simulink model "Path_Flyer"  (R2017b)
settings: Solver=VariableStepAuto  StartTime=0.0  StopTime=500  FixedStep=0.01  MaxStep=0.06  RelTol=1e-3  EnableMultiTasking=on
PreLoadFcn:
  | load('Hummingbird_+.mat');
  | load('Hover_Hum.mat');
StartFcn:
  | clear NLGL
  | clear CARROT
  | clear NLGL_ad_2
  | clear CARROT_ad_2
model workspace (MAT data in the model file):
  Sig = Simulink.Signal
  Sig.DataType = 'auto'
  Sig.Dimensions = -1
  Sig.DimensionsMode = 'auto'
  Sig.Complexity = 'auto'
  Sig.SampleTime = -1
  Sig.SamplingMode = 'auto'
undefined symbols (not defined in the file): IC, quadModel
libraries: simulink x18
Description:
  | This is a configurable quadcopter simulation.
  | This Simulink model demonstates position control.
  | 
  | Additional quadcopter modeling and simulation materials available at:
  | github.com/dch33/Quad-Sim
  | 
  | Copyright (C) 2014 D. Hartman, K. Landis, S. Moreno, J. Kim, M. Mehrer
  | 
  | License:
  |     This program is free software: you can redistribute it and/or modify
  |     it under the terms of the GNU LESSER GENERAL PUBLIC LICENSE as published by
  |     the Free Software Foundation, either version 3 of the License, or
  |     (at your option) any later version.
  | 
  |     This program is distributed in the hope that it will be useful,
  |     but WITHOUT ANY WARRANTY; without even the implied warranty of
  |     MERCHANTABILITY or FITNESS FOR A PARTICULAR PURPOSE.  See the
  |     GNU General Public License for more details.
  | 
  |     You should have received a copy of the GNU LESSER GENERAL PUBLIC LICENSE
  |     along with this program.  If not, see <http://www.gnu.org/licenses/>.
settings Model: ModifiedComment=tomeu -- Fri Oct 14 22:31:49 2016 -- Version 1.12  Creator=David Hartman  LastModifiedBy=tomeu
settings Model: ModifiedHistory=|
  | tomeu -- Fri Oct 14 22:31:49 2016 -- Version 1.12
  | 
  | 
  | tomeu -- Fri Oct 14 22:31:49 2016 -- Version 1.12
  | 
  | 
  | tomeu -- Fri Oct 14 00:32:08 2016 -- Version 1.11
  | 
  | 
  | tomeu -- Thu Oct 13 16:50:12 2016 -- Version 1.10
  | 
  | 
  | tomeu -- Thu Oct 13 14:25:45 2016 -- Version 1.9
  | 
  | 
  | tomeu -- Tue Oct 11 16:42:58 2016 -- Version 1.8
  | 
  | 
  | tomeu -- Mon Oct 10 19:40:14 2016 -- Version 1.7
  | 
  | 
  | tomeu -- Mon Oct 10 16:39:20 2016 -- Version 1.6
  | 
  | 
  | davidhartman -- Fri Jun 06 22:59:54 2014 -- Version 1.5
settings DataIOCC: SaveFormat=Array  SignalLogging=off
settings OptimizationCC: DefaultParameterBehavior=Inlined  LifeSpan=inf
settings DebuggingCC: SolverPrmCheckMsg=warning  UniqueDataStoreMsg=warning  AllowSymbolicDim=off  StateNameClashWarn=warning  StrictBusMsg=ErrorOnBusTreatedAsVector  SFUnexpectedBacktrackingDiag=warning  SFNoUnconditionalDefaultTransitionDiag=warning  SFExecutionAtInitializationDiag=none
settings HardwareCC: ProdBitPerPointer=32  ProdBitPerSizeT=32  ProdBitPerPtrDiffT=32  ProdLargestAtomicFloat=None  ProdIntDivRoundTo=Undefined  ProdEndianess=Unspecified  ProdWordSize=32  ProdHWDeviceType=32-bit Generic
settings ModelReferenceCC: PropagateSignalLabelsOutOfModel=off
settings CodeAppCC: StateflowObjectComments=on
settings GRTTargetCC: TargetLangStandard=C89/C90 (ANSI)  GeneratePreprocessorConditionals=Disable all
settings ConfigComp: CovMetricSettings=dw  CovHtmlReporting=on  CovSaveCumulativeToWorkspaceVar=on  CovSaveSingleToWorkspaceVar=on  CovExternalEMLEnable=off

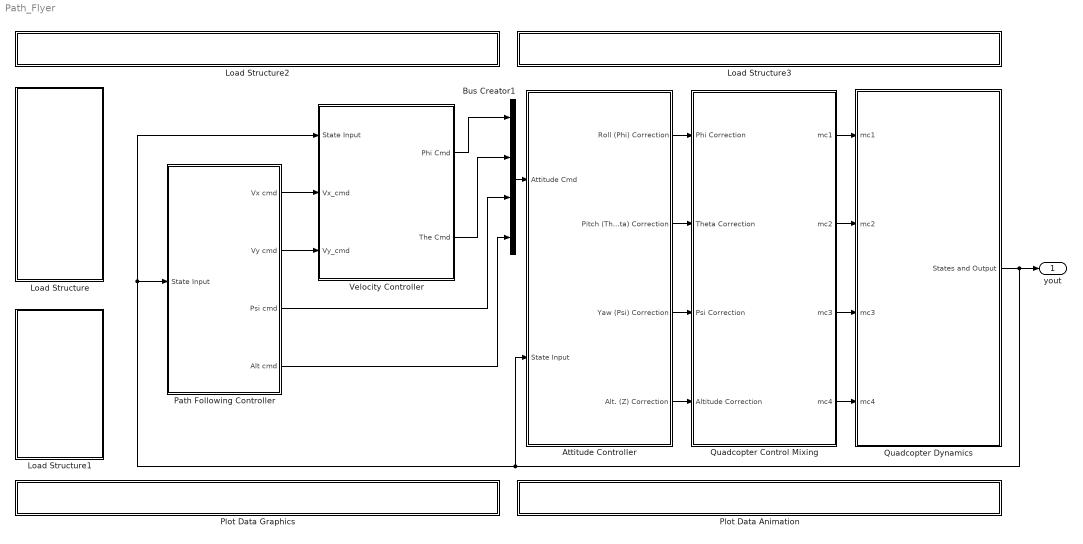
== system Path_Flyer ==
  Attitude Controller : Subsystem
  Bus Creator1 : BusCreator  Inputs=4
  Load Structure : Subsystem
      settings: OpenFcn=|
      | uiopen('load')
      | if ((exist('IC')==1) && (exist('quadModel')==1) && (exist('path')==1))
      | set_param(bdroot, 'SimulationCommand', 'update')
      | end
      mask Display: fprintf('LOAD:\nTimeseries\nPath\nCommands,\nQuadcopter\nModel, Or\nInitial\nConditions');
  Load Structure1 : Subsystem
      settings: OpenFcn=|
      | if (exist('IC')==1 && exist('quadModel')==1 && exist('yout') && exist('tout'))
      | saveSimResults()
      | else
      | msgbox('No Data To Save!')
      | end
      mask Display: fprintf('SAVE:\nSimulation\nResults');
  Load Structure2 : Subsystem
      settings: OpenFcn=|
      | if exist('GUI_Modeling') == 2,
      | run('GUI_Modeling')
      | 
      | else
      | 
      | msgbox('The desired GUI must be first added to MATLABs path.')
      | 
      | end
      mask Display: fprintf('OPEN GUI: Build New \n Model');
  Load Structure3 : Subsystem
      settings: OpenFcn=|
      | if exist('GUI_IC') == 2,
      | run('GUI_IC')
      | 
      | else
      | 
      | msgbox('The desired GUI must be first added to MATLABs path.')
      | 
      | end
      mask Display: fprintf('OPEN GUI: Create Initial \n Conditions');
  Path Following Controller : Subsystem  mask{PF_Algorithm=NLGL, alg_param=1, Adaptive=off, Path_type=Eight-Shaped, Vref=1, A_path=3, gamma_end=1, ZVar=on, Trajplot=on, ErrXplot=off, ErrYplot=off, ErrZplot=off, L2plot=on, YawErrplot=off, Velplot=off, CEffplot=off, AlgParamplot=off, ValueAvgL2=0.18642, ValueAvgYawErr=11.8613, ValueAvgVel=0.97456, ValueAvgCEff=51.0051, ValueTfinal=40.4522}
      mask prompts: alg_param "Algorithm parameter"; Adaptive "Adaptive parameter selection"; Vref "Velocity reference (m/s)"; A_path "Path amplitude (m)"; gamma_end "Path length (turns)"; ZVar "Variable altitude"; Trajplot "3D trajectory"; ErrXplot "Error on X"; ErrYplot "Error on Y"; ErrZplot "Error on Z"; L2plot "Path distance error"; YawErrplot "Yaw angle error"; Velplot "Velocity module"; CEffplot "Control effort"; AlgParamplot "Algorithm parameter"; ValueAvgL2 "Average path distane error (m)"; ValueAvgYawErr "Average absolute yaw error (deg)"; ValueAvgVel "Average absolute velocity (m/s)"; ValueAvgCEff "Average control effort (%)"; ValueTfinal "Total time (s)"
      mask TypeOptions PF_Algorithm: NLGL | Carrot-Chasing
      mask TypeOptions Path_type: Eight-Shaped | Circular | Spiral | Line + Circular
      mask Callback Path_type:
      | Amp_p=str2num(get_param(gcb,'A_path'));
      | load('Hover_Hum.mat');
      | maskStr = get_param(gcb,'Path_type');
      | if strcmp(maskStr,'Eight-Shaped')
      | 	IC.X = IC.X + Amp_p*2;
      |     IC.Psi = IC.Psi + 90;
      | elseif strcmp(maskStr,'Circular')
      | 	IC.X = IC.X + Amp_p;
      |     IC.Psi = IC.Psi + 90;
      | elseif strcmp(maskStr,'Spiral')
      |     IC.Psi = IC.Psi + 90;
      | end
      | 
      | clear maskStr Amp_p;
      mask DialogControl DescGroupVar Prompt: Path Following Control
      mask DialogControl DescTextVar Prompt: This block implements the selected path following algorithm for the desired path command. Parameters such as the velocity of the vehicle, the lenght of the path and the control parameter of the selected algorithm can be changed below.
      mask DialogControl Container5 Prompt: Algorithm
      mask DialogControl Container10 Prompt: Path comand
      mask DialogControl Container3 Prompt: Path Following Evaluation
      mask DialogControl Control4 Prompt: Select which graphs you want to plot and press Run Evaluation button.
      mask DialogControl Container7 Prompt: Plots
      mask DialogControl Container9 Prompt: Results
      mask DialogControl RunEvaluation Prompt: Run Evaluation
      mask DialogControl RunEvaluation Callback:
      | maskStr = get_param(gcb,'Path_type');
      | if strcmp(maskStr,'Eight-Shaped')
      |     path_type = 1;
      | elseif strcmp(maskStr,'Circular')
      |     path_type = 2;
      | elseif strcmp(maskStr,'Spiral')
      |     path_type = 3;
      | elseif strcmp(maskStr,'Line + Circular')
      |     path_type = 4;
      | end
      | 
      | if strcmp(get_param(gcb,'ZVar'),'on')
      |     z_var = 1;
      | else
      |     z_var = 0;
      | end
      | g_end=str2num(get_param(gcb,'gamma_end'));
      | 
      | Amp_path=str2num(get_param(gcb,'A_path'));
      | 
      | Traj_plot = get_param(gcb,'Trajplot');
      | ErrX_plot = get_param(gcb,'ErrXplot');
      | ErrY_plot = get_param(gcb,'ErrYplot');
      | ErrZ_plot = get_param(gcb,'ErrZplot');
      | L2_plot = get_param(gcb,'L2plot');
      | YawErr_plot = get_param(gcb,'YawErrplot');
      | Vel_plot = get_param(gcb,'Velplot');
      | CEff_plot = get_param(gcb,'CEffplot');
      | AlgParam_plot = get_param(gcb,'AlgParamplot');
      | 
      | analyse;
      | 
      | set_param(gcb,'ValueAvgL2',num2str(meanL2_3D));
      | set_param(gcb,'ValueAvgYawErr',num2str(meanAbsYawErr));
      | set_param(gcb,'ValueAvgVel',num2str(meanVel));
      | set_param(gcb,'ValueAvgCEff',num2str(meanCEffort));
      | set_param(gcb,'ValueTfinal',num2str(Tfinal));
      | 
      | clear maskStr path_type Traj_plot ErrX_plot ErrY_plot ErrZ_plot;
      | clear L2_plot YawErr_plot Vel_plot CEff_plot AlgParam_plot g_end z_var;
      | clear meanL2_3D meanAbsYawErr meanVel meanCEffort Tfinal
  Plot Data Animation : Subsystem
      settings: OpenFcn=|
      | if exist('QuadAnim4') == 2,
      |     if exist('yout')
      | 	run('QuadAnim4');
      |     else
      |     msgbox('Simulation must be run before data can be plotted.');
      |     end
      | else                                                                          msgbox('The desired GUI must be first added to MATLABs path.')
      | end
      mask Display: fprintf('OPEN GUI: Flight Animation')
  Plot Data Graphics : Subsystem
      settings: OpenFcn=|
      | if exist('yout')
      | yout = evalin('base', 'yout');
      | tout = evalin('base', 'tout');
      | quadPlots(yout, tout)
      | else
      | msgbox('Simulation must be run before data can be plotted.')
      | end
      mask Display: fprintf('OPEN PLOT: State Data')
  Quadcopter Control Mixing : Subsystem
      mask Display:
      | modelLoaded = evalin('base','exist(''quadModel'',''var'')');
      | if (modelLoaded==1)
      |     if (evalin('base','quadModel.plusConfig'))
      |     fprintf([' \n' ' \n'  'Configuration "+"']);
      |     else if (~evalin('base','quadModel.plusConfig'))
      |         fprintf([' \n' ' \n' 'Configuration "X"']);
      |         end
      |     end
      | else
      |     fprintf([' \n' ' \n'  'Model Not Loaded']);
      | end
  Quadcopter Dynamics : Subsystem
  Velocity Controller : Subsystem
  yout : Outport
  wires:
  Quadcopter Control Mixing/1(mc1) -> Quadcopter Dynamics/1(mc1)
  Quadcopter Control Mixing/2(mc2) -> Quadcopter Dynamics/2(mc2)
  Quadcopter Control Mixing/3(mc3) -> Quadcopter Dynamics/3(mc3)
  Quadcopter Control Mixing/4(mc4) -> Quadcopter Dynamics/4(mc4)
  Attitude Controller/1(Roll (Phi) Correction) -> Quadcopter Control Mixing/1(Phi Correction)
  Attitude Controller/2(Pitch (Theta) Correction) -> Quadcopter Control Mixing/2(Theta Correction)
  Attitude Controller/3(Yaw (Psi) Correction) -> Quadcopter Control Mixing/3(Psi Correction)
  Attitude Controller/4(Alt. (Z) Correction) -> Quadcopter Control Mixing/4(Altitude Correction)
  Quadcopter Dynamics/1(States and Output) -> yout/1, Velocity Controller/1(State Input), Path Following Controller/1(State Input), Attitude Controller/2(State Input)
  Bus Creator1/1 -> Attitude Controller/1(Attitude Cmd)
  Path Following Controller/3(Psi cmd) -> Bus Creator1/3
  Path Following Controller/4(Alt cmd) -> Bus Creator1/4
  Velocity Controller/1(Phi Cmd) -> Bus Creator1/1
  Velocity Controller/2(The Cmd) -> Bus Creator1/2
  Path Following Controller/2(Vy cmd) -> Velocity Controller/3(Vy_cmd)
  Path Following Controller/1(Vx cmd) -> Velocity Controller/2(Vx_cmd)

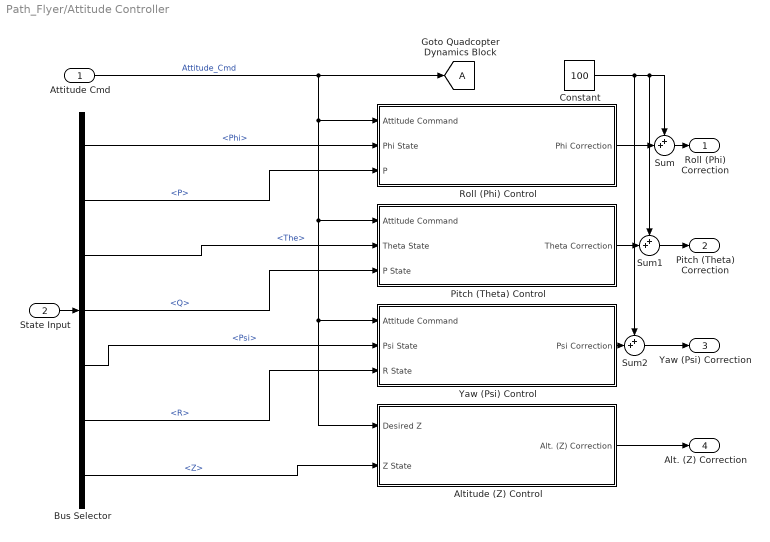
== system Path_Flyer/Attitude Controller ==
  Attitude Cmd : Inport
  State Input : Inport  Port=2
  Altitude (Z) Control : Subsystem  mask{Kpz=2*2, Kiz=1.1*2, Kdz=3.3*2, LimitOutput=on, USat=1, LSat=-1, GOffset=(sqrt((quadModel.mass*quadModel.g)/(4*quadModel.ct))-quadModel.b)/quadModel.cr}
      mask prompts: Kpz "Kp"; Kiz "Ki"; Kdz "Kd"; LimitOutput "Integral Saturation?"; USat "Upper saturation limit:"; LSat "Lower saturation limit:"; GOffset "Gravity Feedforward"
      mask help:
      | Adjust PID controller gains through this mask interface, or "look under mask" for more detailed adjustments.
      |
      | Note: Gravity Offset will not appear on block face as a value until simulation is run if it is the result of a formula involving the quadcopter model parameters.
      mask TypeOptions Kpz: Kpz/Gain
      mask TypeOptions Kiz: Kiz/Gain
      mask TypeOptions Kdz: Kdz/Gain
      mask TypeOptions LimitOutput:
      | Integrator
      | Limited/LimitOutput
      mask TypeOptions USat:
      | Integrator
      | Limited/UpperSaturationLimit
      mask TypeOptions LSat:
      | Integrator
      | Limited/LowerSaturationLimit
      mask TypeOptions GOffset: Gravity Offset (Level Flight)/Value
      mask Display:
      | fprintf(['Gravity Offset = ' num2str(GOffset) '\n' ...
      |     'Kp = ' num2str(Kpz) '\n' ...
      |     'Ki = ' num2str(Kiz) '\n' ...
      |     'Kd = ' num2str(Kdz) '\n' ...
      |     'Integral Saturation: ' LimitOutput]);
      | if strcmp(LimitOutput,'on')
      |     fprintf([' \n' ' \n' ' \n' ' \n' ' \n' '\n' ...
      |         'Limits: ' num2str(USat) ' to ' num2str(LSat)]);
      | end
  Bus Selector : BusSelector  OutputSignals=Phi,P,The,Q,Psi,R,Z
  Constant : Constant  Value=100
  Pitch (Theta) Control : Subsystem  mask{Kpt=2*2, Kit=1.1*2, Kdt=1.2*2, LimitOutput=on, USat=100, LSat=-100}
      mask prompts: Kpt "Kp"; Kit "Ki"; Kdt "Kd"; LimitOutput "Integral Saturation?"; USat "Upper saturation limit:"; LSat "Lower saturation limit:"
      mask help: Adjust PID controller gains through this mask interface, or "look under mask" for more detailed adjustments.
      mask TypeOptions Kpt: Kpt/Gain
      mask TypeOptions Kit: Kit/Gain
      mask TypeOptions Kdt: Kdt/Gain
      mask TypeOptions LimitOutput:
      | Integrator
      | Limited/LimitOutput
      mask TypeOptions USat:
      | Integrator
      | Limited/UpperSaturationLimit
      mask TypeOptions LSat:
      | Integrator
      | Limited/LowerSaturationLimit
      mask Display:
      | fprintf(['Kp = ' num2str(Kpt) '\n' ...
      |     'Ki = ' num2str(Kit) '\n' ...
      |     'Kd = ' num2str(Kdt) '\n' ...
      |     'Integral Saturation: ' LimitOutput]);
      | if strcmp(LimitOutput,'on')
      |     fprintf([' \n' ' \n' ' \n' ' \n' '\n' ...
      |         'Limits: ' num2str(USat) ' to ' num2str(LSat)]);
      | end
  "Roll (Phi) Control " : Subsystem  mask{Kpp=2.0*2, Kip=1.1*2, Kdp=1.2*2, LimitOutput=on, USat=100, LSat=-100}
      mask prompts: Kpp "Kp"; Kip "Ki"; Kdp "Kd"; LimitOutput "Integral Saturation:"; USat "Upper saturation limit:"; LSat "Lower saturation limit:"
      mask help:
      | Adjust PID controller gains through this mask interface, or "look under mask"
      | for more detailed adjustments.
      mask TypeOptions Kpp: Kpp/Gain
      mask TypeOptions Kip: Kip/Gain
      mask TypeOptions Kdp: Kdp/Gain
      mask TypeOptions LimitOutput:
      | Integrator
      | Limited/LimitOutput
      mask TypeOptions USat:
      | Integrator
      | Limited/UpperSaturationLimit
      mask TypeOptions LSat:
      | Integrator
      | Limited/LowerSaturationLimit
      mask Display:
      | fprintf(['Kp = ' num2str(Kpp) '\n' ...
      |     'Ki = ' num2str(Kip) '\n' ...
      |     'Kd = ' num2str(Kdp) '\n'...
      |     'Integral Saturation: ' LimitOutput]);
      | if strcmp(LimitOutput,'on')
      |     fprintf([' \n' ' \n' ' \n' ' \n' '\n' ...
      |         'Limits: ' num2str(USat) ' to ' num2str(LSat)]);
      | end
  Sum : Sum  Inputs=++|
  Sum1 : Sum  Inputs=++|
  Sum2 : Sum  Inputs=++|
  Yaw (Psi) Control : Subsystem  mask{Kps=4*2, Kis=0.5*2, Kds=3.5*2, LimitOutput=on, USat=1, LSat=-1}
      mask prompts: Kps "Kp"; Kis "Ki"; Kds "Kd"; LimitOutput "Integral Saturation?"; USat "Upper saturation limit:"; LSat "Lower saturation limit:"
      mask help: Adjust PID controller gains through this mask interface, or "look under mask" for more detailed adjustments.
      mask TypeOptions Kps: Kps/Gain
      mask TypeOptions Kis: Kit/Gain
      mask TypeOptions Kds: Kds/Gain
      mask TypeOptions LimitOutput:
      | Integrator
      | Limited/LimitOutput
      mask TypeOptions USat:
      | Integrator
      | Limited/UpperSaturationLimit
      mask TypeOptions LSat:
      | Integrator
      | Limited/LowerSaturationLimit
      mask Display:
      | fprintf(['Kp = ' num2str(Kps) '\n' ...
      |     'Ki = ' num2str(Kis) '\n' ...
      |     'Kd = ' num2str(Kds) '\n' ...
      |     'Integral Saturation: ' LimitOutput]);
      | if strcmp(LimitOutput,'on')
      |     fprintf([' \n' ' \n' ' \n' ' \n' '\n' ...
      |         'Limits: ' num2str(USat) ' to ' num2str(LSat)]);
      | end
  Roll (Phi) Correction : Outport
  Pitch (Theta) Correction : Outport  Port=2
  Yaw (Psi) Correction : Outport  Port=3
  Alt. (Z) Correction : Outport  Port=4
  tag scope: A=global
  wires:
  State Input/1 -> Bus Selector/1
  Bus Selector/5 -> Yaw (Psi) Control/2(Psi State)  "<Psi>"
  Bus Selector/7 -> Altitude (Z) Control/2(Z State)  "<Z>"
  Bus Selector/2 -> "Roll (Phi) Control "/3(P)  "<P>"
  Bus Selector/4 -> Pitch (Theta) Control/3(P State)  "<Q>"
  Bus Selector/6 -> Yaw (Psi) Control/3(R State)  "<R>"
  Attitude Cmd/1 -> [A], Altitude (Z) Control/1(Desired Z), Yaw (Psi) Control/1(Attitude Command), Pitch (Theta) Control/1(Attitude Command), "Roll (Phi) Control "/1("Attitude Command ")  "Attitude_Cmd"
  Altitude (Z) Control/1(Alt. (Z) Correction) -> Alt. (Z) Correction/1
  Bus Selector/1 -> "Roll (Phi) Control "/2(Phi State)  "<Phi>"
  Bus Selector/3 -> Pitch (Theta) Control/2(Theta State)  "<The>"
  "Roll (Phi) Control "/1(Phi Correction) -> Sum/2
  Sum/1 -> Roll (Phi) Correction/1
  Sum1/1 -> Pitch (Theta) Correction/1
  Pitch (Theta) Control/1(Theta Correction) -> Sum1/2
  Sum2/1 -> Yaw (Psi) Correction/1
  Yaw (Psi) Control/1(Psi Correction) -> Sum2/2
  Constant/1 -> Sum2/1, Sum1/1, Sum/1

== system Path_Flyer/Load Structure ==

== system Path_Flyer/Load Structure1 ==

== system Path_Flyer/Load Structure2 ==

== system Path_Flyer/Load Structure3 ==

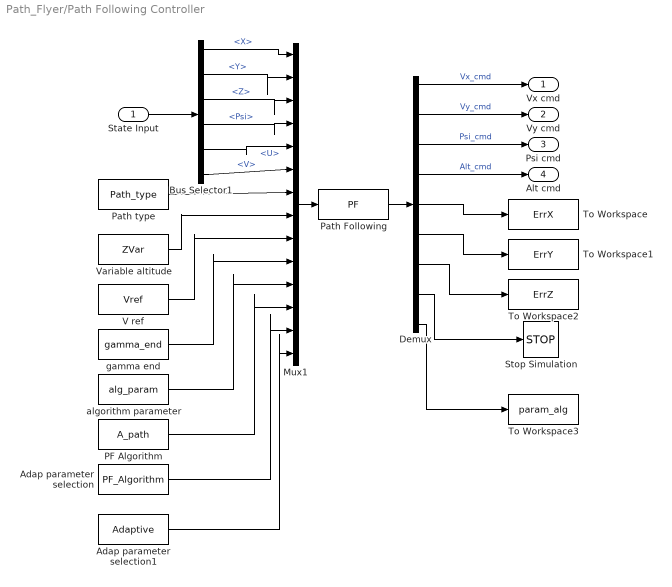
== system Path_Flyer/Path Following Controller ==
  State Input : Inport
  Adap parameter selection : Constant  Value=PF_Algorithm
  Adap parameter selection1 : Constant  Value=Adaptive
  Bus Selector1 : BusSelector  OutputSignals=X,Y,Z,Psi,U,V
  Demux : Demux  Outputs=9
  Mux1 : Mux  Inputs=14
  PF Algorithm : Constant  Value=A_path
  Path Following : MATLABFcn  MATLABFcn=PF  OutputDimensions=9
  Path type : Constant  Value=Path_type
  Stop Simulation : Stop
  To Workspace : ToWorkspace  VariableName=ErrX  SaveFormat=Timeseries  SampleTime=-1
  To Workspace1 : ToWorkspace  VariableName=ErrY  SaveFormat=Timeseries  SampleTime=-1
  To Workspace2 : ToWorkspace  VariableName=ErrZ  SaveFormat=Timeseries  SampleTime=-1
  To Workspace3 : ToWorkspace  VariableName=param_alg  SaveFormat=Timeseries  SampleTime=-1
  V ref : Constant  Value=Vref
  Variable altitude : Constant  Value=ZVar
  algorithm parameter : Constant  Value=alg_param
  gamma end : Constant  Value=gamma_end
  Vx cmd : Outport
  Vy cmd : Outport  Port=2
  Psi cmd : Outport  Port=3
  Alt cmd : Outport  Port=4
  wires:
  Bus Selector1/2 -> Mux1/2  "<Y>"
  Bus Selector1/4 -> Mux1/4  "<Psi>"
  Bus Selector1/1 -> Mux1/1  "<X>"
  Path Following/1 -> Demux/1
  Mux1/1 -> Path Following/1
  Bus Selector1/3 -> Mux1/3  "<Z>"
  State Input/1 -> Bus Selector1/1
  Demux/4 -> Alt cmd/1  "Alt_cmd"
  Demux/3 -> Psi cmd/1  "Psi_cmd"
  Demux/1 -> Vx cmd/1  "Vx_cmd"
  Demux/2 -> Vy cmd/1  "Vy_cmd"
  Demux/5 -> To Workspace/1
  Demux/6 -> To Workspace1/1
  Demux/8 -> Stop Simulation/1
  Demux/7 -> To Workspace2/1
  Bus Selector1/5 -> Mux1/5  "<U>"
  Bus Selector1/6 -> Mux1/6  "<V>"
  Path type/1 -> Mux1/7
  Demux/9 -> To Workspace3/1
  Variable altitude/1 -> Mux1/8
  V ref/1 -> Mux1/9
  gamma end/1 -> Mux1/10
  algorithm parameter/1 -> Mux1/11
  PF Algorithm/1 -> Mux1/12
  Adap parameter selection/1 -> Mux1/13
  Adap parameter selection1/1 -> Mux1/14

== system Path_Flyer/Plot Data Animation ==

== system Path_Flyer/Plot Data Graphics ==

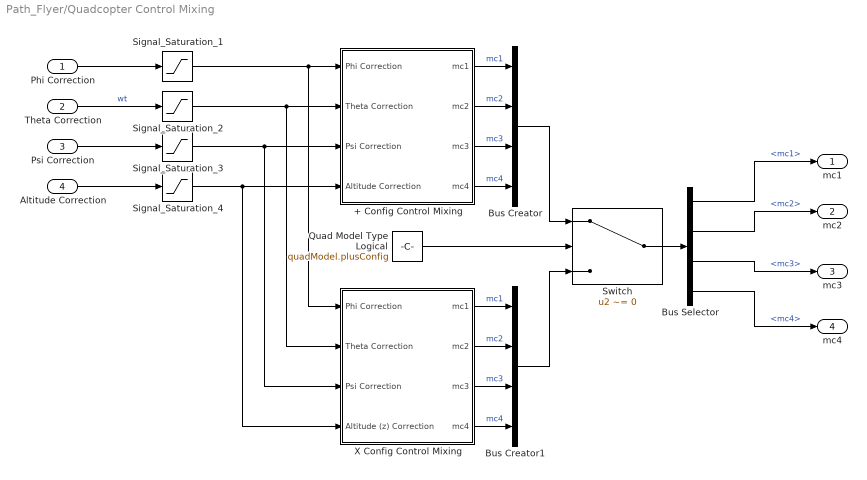
== system Path_Flyer/Quadcopter Control Mixing ==
  Phi Correction : Inport
  Theta Correction : Inport  Port=2
  Psi Correction : Inport  Port=3
  Altitude Correction : Inport  Port=4
  + Config Control Mixing : Subsystem
  Bus Creator : BusCreator  Inputs=4
  Bus Creator1 : BusCreator  Inputs=4
  Bus Selector : BusSelector  OutputSignals=mc1,mc2,mc3,mc4
  Quad Model Type Logical : Constant  Value=quadModel.plusConfig
  Signal_Saturation_{1..4} (4 alike) : Saturate  UpperLimit=200  LowerLimit=0
  Switch : Switch  Criteria=u2 ~= 0
  X Config Control Mixing : Subsystem
  mc1 : Outport
  mc2 : Outport  Port=2
  mc3 : Outport  Port=3
  mc4 : Outport  Port=4
  wires:
  Phi Correction/1 -> Signal_Saturation_1/1
  Theta Correction/1 -> Signal_Saturation_2/1  "wt"
  Psi Correction/1 -> Signal_Saturation_3/1
  + Config Control Mixing/1(mc1) -> Bus Creator/1  "mc1"
  + Config Control Mixing/2(mc2) -> Bus Creator/2  "mc2"
  + Config Control Mixing/3(mc3) -> Bus Creator/3  "mc3"
  + Config Control Mixing/4(mc4) -> Bus Creator/4  "mc4"
  Bus Creator/1 -> Switch/1
  X Config Control Mixing/1(mc1) -> Bus Creator1/1  "mc1"
  X Config Control Mixing/2(mc2) -> Bus Creator1/2  "mc2"
  X Config Control Mixing/3(mc3) -> Bus Creator1/3  "mc3"
  X Config Control Mixing/4(mc4) -> Bus Creator1/4  "mc4"
  Bus Creator1/1 -> Switch/3
  Bus Selector/1 -> mc1/1  "<mc1>"
  Bus Selector/2 -> mc2/1  "<mc2>"
  Bus Selector/3 -> mc3/1  "<mc3>"
  Bus Selector/4 -> mc4/1  "<mc4>"
  Quad Model Type Logical/1 -> Switch/2
  Switch/1 -> Bus Selector/1
  Altitude Correction/1 -> Signal_Saturation_4/1
  Signal_Saturation_1/1 -> X Config Control Mixing/1(Phi Correction), + Config Control Mixing/1(Phi Correction)
  Signal_Saturation_2/1 -> X Config Control Mixing/2(Theta Correction), + Config Control Mixing/2(Theta Correction)
  Signal_Saturation_3/1 -> X Config Control Mixing/3(Psi Correction), + Config Control Mixing/3(Psi Correction)
  Signal_Saturation_4/1 -> X Config Control Mixing/4(Altitude (z) Correction), + Config Control Mixing/4(Altitude Correction)

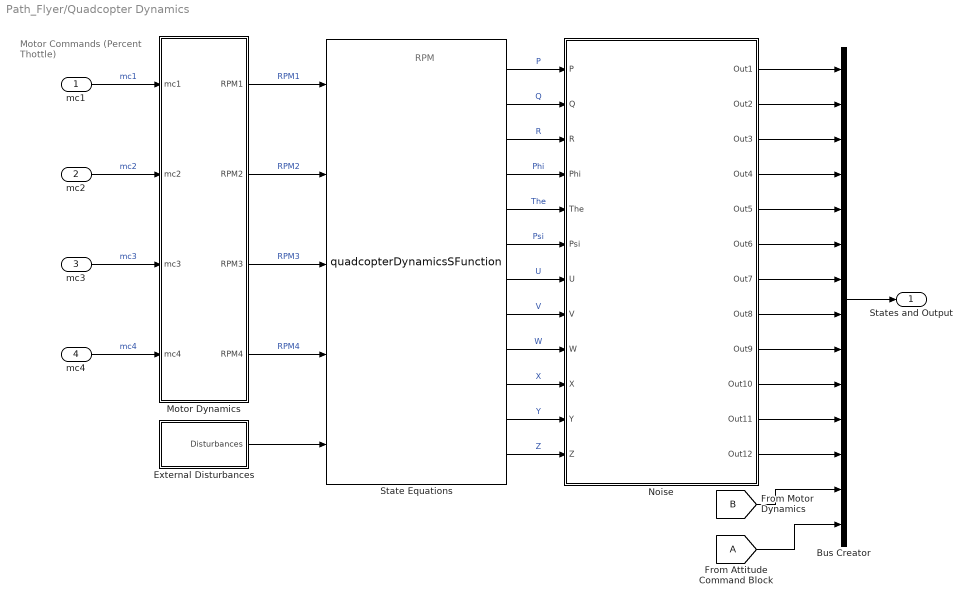
== system Path_Flyer/Quadcopter Dynamics ==
  note: RPM
  note: Motor Commands
      | (Percent Thottle)
  mc1 : Inport
  mc2 : Inport  Port=2
  mc3 : Inport  Port=3
  mc4 : Inport  Port=4
  Bus Creator : BusCreator  Inputs='P','Q','R','Phi','The','Psi','U','V','W','X','Y','Z','mc and RPM','Attitude_Cmd'
  External Disturbances : Subsystem
  Motor Dynamics : Subsystem
  Noise : Subsystem
  State Equations : M-S-Function  FunctionName=quadcopterDynamicsSFunction  Parameters=quadModel, IC
      mask Display:
      | port_label('input', 1, 'RPM1')
      | port_label('input', 2, 'RPM2')
      | port_label('input', 3, 'RPM3')
      | port_label('input', 4, 'RPM4')
      | port_label('input', 5, 'Disturbances')
      | port_label('output', 1, 'P')
      | port_label('output', 2, 'Q')
      | port_label('output', 3, 'R')
      | port_label('output', 4, 'Phi')
      | port_label('output', 5, 'The')
      | port_label('output', 6, 'Psi')
      | port_label('output', 7, 'U')
      | port_label('output', 8, 'V')
      | port_label('output', 9, 'W')
      | port_label('output', 10, 'X')
      | port_label('output', 11, 'Y')
      | port_label('output', 12, 'Z')
  States and Output : Outport
  wires:
  Bus Creator/1 -> States and Output/1
  Motor Dynamics/1(RPM1) -> State Equations/1  "RPM1"
  Motor Dynamics/2(RPM2) -> State Equations/2  "RPM2"
  Motor Dynamics/3(RPM3) -> State Equations/3  "RPM3"
  Motor Dynamics/4(RPM4) -> State Equations/4  "RPM4"
  mc1/1 -> Motor Dynamics/1(mc1)  "mc1"
  mc4/1 -> Motor Dynamics/4(mc4)  "mc4"
  mc3/1 -> Motor Dynamics/3(mc3)  "mc3"
  mc2/1 -> Motor Dynamics/2(mc2)  "mc2"
  External Disturbances/1("Disturbances ") -> State Equations/5
  [A] -> Bus Creator/14
  [B] -> Bus Creator/13
  State Equations/1 -> Noise/1(P)  "P"
  Noise/1(Out1) -> Bus Creator/1
  Noise/2(Out2) -> Bus Creator/2
  Noise/3(Out3) -> Bus Creator/3
  Noise/4(Out4) -> Bus Creator/4
  Noise/6(Out6) -> Bus Creator/6
  Noise/8(Out8) -> Bus Creator/8
  Noise/5(Out5) -> Bus Creator/5
  Noise/7(Out7) -> Bus Creator/7
  Noise/9(Out9) -> Bus Creator/9
  Noise/10(Out10) -> Bus Creator/10
  Noise/11(Out11) -> Bus Creator/11
  Noise/12(Out12) -> Bus Creator/12
  State Equations/12 -> Noise/12(Z)  "Z"
  State Equations/11 -> Noise/11(Y)  "Y"
  State Equations/2 -> Noise/2(Q)  "Q"
  State Equations/3 -> Noise/3(R)  "R"
  State Equations/4 -> Noise/4(Phi)  "Phi"
  State Equations/5 -> Noise/5(The)  "The"
  State Equations/6 -> Noise/6(Psi)  "Psi"
  State Equations/7 -> Noise/7(U)  "U"
  State Equations/8 -> Noise/8(V)  "V"
  State Equations/9 -> Noise/9(W)  "W"
  State Equations/10 -> Noise/10(X)  "X"

== system Path_Flyer/Velocity Controller ==
  note: Inertial-frame velocity is used as the state to be controlled,
      | (as this is what is controlled by attitude)
      | thus we find position error in the body frame
      | and map this to a body frame desired velocity. This desired
      | velocity is then mapped to a desired attitude.
  State Input : Inport
  Vx_cmd : Inport  Port=2
  Vy_cmd : Inport  Port=3
  Bus Selector1 : BusSelector  OutputSignals=V,U
  Phi Command Control : Subsystem  mask{Kp=0.32, Kd=0.1, ASat=45*pi/180}
      mask prompts: Kp "Proportional Gain"; Kd "Derivative Gain"; ASat "Attitude Limit (+/- radians):"
      mask TypeOptions Kp: Kpp/Gain
      mask TypeOptions Kd: Kdp/Gain
      mask TypeOptions ASat: Attitude Limits_Phi/UpperLimit
      mask Display:
      | fprintf(['Kp = ' num2str(Kp) '\n' ...
      |     'Kd = ' num2str(Kd) '\n' ...
      |     'Attitude Limit (+/-): ' num2str(ASat*180/pi) '°']);
  Theta Command Control : Subsystem  mask{Kp=0.32, Kd=0.10, ASat=45*pi/180}
      mask prompts: Kp "Proportional Gain:"; Kd "Derivative Gain"; ASat "Attitude Limit (+/- radians):"
      mask TypeOptions Kp: Kpt/Gain
      mask TypeOptions Kd: Kdt/Gain
      mask TypeOptions ASat: Attitude Limits_Theta/UpperLimit
      mask Display:
      | fprintf(['Kp = ' num2str(Kp) '\n' ...
      |     'Kd = ' num2str(Kd) '\n' ...
      |     'Attitude Limit (+/-): ' num2str(ASat*180/pi) '°']);
  Phi Cmd : Outport
  The Cmd : Outport  Port=2
  wires:
  State Input/1 -> Bus Selector1/1
  Phi Command Control/1(Phi_cmd) -> Phi Cmd/1  "Phi_Cmd"
  Vx_cmd/1 -> Theta Command Control/1(Desired Xb Velocity)  "Desired velocity in Xb"
  Vy_cmd/1 -> Phi Command Control/1(Desired Yb Velocity)  "Desired Velocity in Yb"
  Bus Selector1/2 -> Theta Command Control/2(Xb Velocity)  "<U>"
  Bus Selector1/1 -> Phi Command Control/2(Yb Velocity)  "<V>"
  Theta Command Control/1(The_cmd) -> The Cmd/1  "The_cmd"

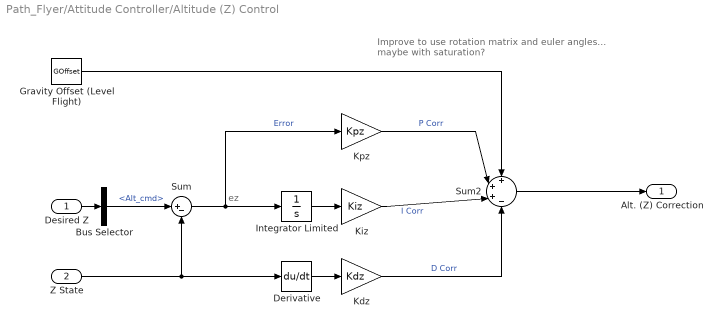
== system Path_Flyer/Attitude Controller/Altitude (Z) Control ==
  note: Improve to use rotation matrix and euler angles...
      | maybe with saturation?
  note: ez
  Desired Z : Inport
  Z State : Inport  Port=2
  Bus Selector : BusSelector  OutputSignals=Alt_cmd
  Derivative : Derivative
  Gravity Offset (Level Flight) : Constant  Value=GOffset
  Integrator Limited : Integrator  LimitOutput=on  UpperSaturationLimit=USat  LowerSaturationLimit=LSat
  Kdz : Gain  Gain=Kdz
  Kiz : Gain  Gain=Kiz
  Kpz : Gain  Gain=Kpz
  Sum : Sum  Inputs=|+-
  Sum2 : Sum  Inputs=+++-
  Alt. (Z) Correction : Outport
  wires:
  Gravity Offset (Level Flight)/1 -> Sum2/1
  Desired Z/1 -> Bus Selector/1
  Z State/1 -> Derivative/1, Sum/2
  Sum2/1 -> Alt. (Z) Correction/1
  Kpz/1 -> Sum2/2  "P Corr"
  Sum/1 -> Integrator Limited/1, Kpz/1  "Error"
  Kiz/1 -> Sum2/3  "I Corr"
  Kdz/1 -> Sum2/4  "D Corr"
  Integrator Limited/1 -> Kiz/1
  Bus Selector/1 -> Sum/1  "<Alt_cmd>"
  Derivative/1 -> Kdz/1

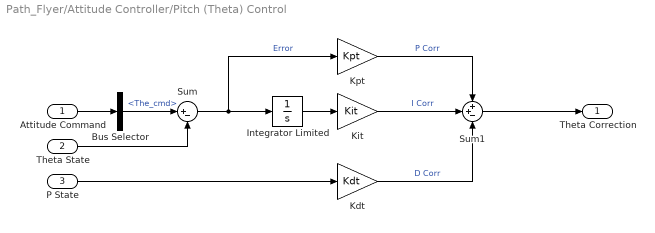
== system Path_Flyer/Attitude Controller/Pitch (Theta) Control ==
  Attitude Command : Inport
  Theta State : Inport  Port=2
  P State : Inport  Port=3
  Bus Selector : BusSelector  OutputSignals=The_cmd
  Integrator Limited : Integrator  LimitOutput=on  UpperSaturationLimit=USat  LowerSaturationLimit=LSat
  Kdt : Gain  Gain=Kdt
  Kit : Gain  Gain=Kit
  Kpt : Gain  Gain=Kpt
  Sum : Sum  Inputs=|+-
  Sum1 : Sum  Inputs=++-
  Theta Correction : Outport
  wires:
  Sum/1 -> Integrator Limited/1, Kpt/1  "Error"
  Attitude Command/1 -> Bus Selector/1
  Theta State/1 -> Sum/2
  Sum1/1 -> Theta Correction/1
  Kpt/1 -> Sum1/1  "P Corr"
  Kdt/1 -> Sum1/3  "D Corr"
  Kit/1 -> Sum1/2  "I Corr"
  Integrator Limited/1 -> Kit/1
  Bus Selector/1 -> Sum/1  "<The_cmd>"
  P State/1 -> Kdt/1

== system Path_Flyer/Attitude Controller/Roll (Phi) Control  ==
  "Attitude Command " : Inport
  Phi State : Inport  Port=2
  P : Inport  Port=3
  Bus Selector : BusSelector  OutputSignals=Phi_Cmd
  Integrator Limited : Integrator  LimitOutput=on  UpperSaturationLimit=USat  LowerSaturationLimit=LSat
  Kdp : Gain  Gain=Kdp
  Kip : Gain  Gain=Kip
  Kpp : Gain  Gain=Kpp
  Sum : Sum  Inputs=|+-
  Sum1 : Sum  Inputs=++-
  Phi Correction : Outport
  wires:
  Sum/1 -> Integrator Limited/1, Kpp/1  "Error"
  Phi State/1 -> Sum/2
  Sum1/1 -> Phi Correction/1
  Kpp/1 -> Sum1/1  "P Corr"
  Kdp/1 -> Sum1/3  "D Corr"
  Kip/1 -> Sum1/2  "I Corr"
  Integrator Limited/1 -> Kip/1
  "Attitude Command "/1 -> Bus Selector/1
  Bus Selector/1 -> Sum/1  "<Phi_Cmd>"
  P/1 -> Kdp/1

== system Path_Flyer/Attitude Controller/Yaw (Psi) Control ==
  Attitude Command : Inport
  Psi State : Inport  Port=2
  R State : Inport  Port=3
  Bus Selector : BusSelector  OutputSignals=Psi_cmd
  Integrator Limited : Integrator  LimitOutput=on  UpperSaturationLimit=USat  LowerSaturationLimit=LSat
  Kds : Gain  Gain=Kds
  Kit : Gain  Gain=Kis
  Kps : Gain  Gain=Kps
  Sum : Sum  Inputs=|+-
  Sum1 : Sum  Inputs=++-
  Psi Correction : Outport
  wires:
  Sum/1 -> Integrator Limited/1, Kps/1  "Error"
  Attitude Command/1 -> Bus Selector/1
  Sum1/1 -> Psi Correction/1
  Psi State/1 -> Sum/2
  Kps/1 -> Sum1/1  "P Corr"
  Kds/1 -> Sum1/3  "D Corr"
  Kit/1 -> Sum1/2  "I Corr"
  Integrator Limited/1 -> Kit/1
  Bus Selector/1 -> Sum/1  "<Psi_cmd>"
  R State/1 -> Kds/1

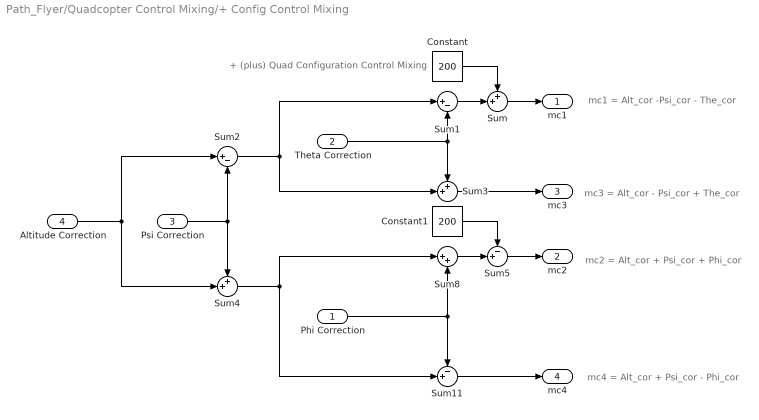
== system Path_Flyer/Quadcopter Control Mixing/+ Config Control Mixing ==
  note: mc2 = Alt_cor + Psi_cor + Phi_cor
  note: + (plus) Quad Configuration Control Mixing
  note: mc4 = Alt_cor + Psi_cor - Phi_cor
  note: mc3 = Alt_cor - Psi_cor + The_cor
  note: mc1 = Alt_cor -Psi_cor - The_cor
  Phi Correction : Inport
  Theta Correction : Inport  Port=2
  Psi Correction : Inport  Port=3
  Altitude Correction : Inport  Port=4
  Constant : Constant  Value=200
  Constant1 : Constant  Value=200
  Sum : Sum  Inputs=++|
  Sum1 : Sum  Inputs=|+-
  Sum11 : Sum  Inputs=-+|
  Sum2 : Sum  Inputs=|+-
  Sum3 : Sum  Inputs=++|
  Sum4 : Sum  Inputs=++|
  Sum5 : Sum  Inputs=-+|
  Sum8 : Sum  Inputs=|++
  mc1 : Outport
  mc2 : Outport  Port=2
  mc3 : Outport  Port=3
  mc4 : Outport  Port=4
  wires:
  Theta Correction/1 -> Sum1/2, Sum3/1
  Altitude Correction/1 -> Sum2/1, Sum4/2
  Sum2/1 -> Sum3/2, Sum1/1
  Psi Correction/1 -> Sum4/1, Sum2/2
  Sum4/1 -> Sum11/2, Sum8/1
  Phi Correction/1 -> Sum8/2, Sum11/1
  Sum3/1 -> mc3/1
  Sum11/1 -> mc4/1
  Sum/1 -> mc1/1
  Sum1/1 -> Sum/2
  Sum5/1 -> mc2/1
  Sum8/1 -> Sum5/2
  Constant/1 -> Sum/1
  Constant1/1 -> Sum5/1

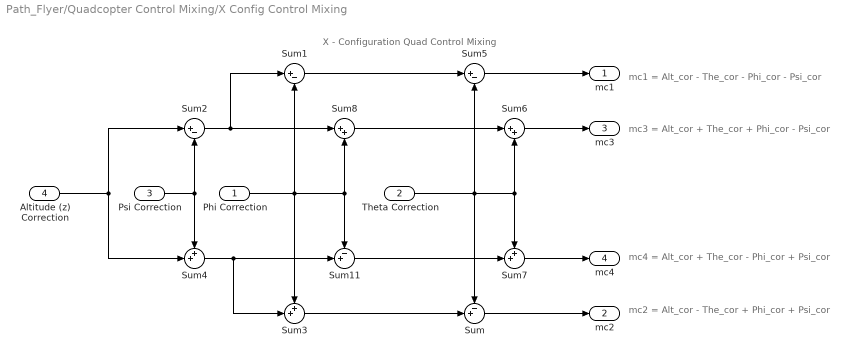
== system Path_Flyer/Quadcopter Control Mixing/X Config Control Mixing ==
  note: mc1 = Alt_cor - The_cor - Phi_cor - Psi_cor
  note: X - Configuration Quad Control Mixing
  note: mc3 = Alt_cor + The_cor + Phi_cor - Psi_cor
  note: mc2 = Alt_cor - The_cor + Phi_cor + Psi_cor
  note: mc4 = Alt_cor + The_cor - Phi_cor + Psi_cor
  Phi Correction : Inport
  Theta Correction : Inport  Port=2
  Psi Correction : Inport  Port=3
  Altitude (z) Correction : Inport  Port=4
  Sum : Sum  Inputs=-+|
  Sum1 : Sum  Inputs=|+-
  Sum11 : Sum  Inputs=-+|
  Sum2 : Sum  Inputs=|+-
  Sum3 : Sum  Inputs=++|
  Sum4 : Sum  Inputs=++|
  Sum5 : Sum  Inputs=|+-
  Sum6 : Sum  Inputs=|++
  Sum7 : Sum  Inputs=++|
  Sum8 : Sum  Inputs=|++
  mc1 : Outport
  mc2 : Outport  Port=2
  mc3 : Outport  Port=3
  mc4 : Outport  Port=4
  wires:
  Sum2/1 -> Sum8/1, Sum1/1
  Psi Correction/1 -> Sum4/1, Sum2/2
  Phi Correction/1 -> Sum3/1, Sum1/2, Sum8/2, Sum11/1
  Sum4/1 -> Sum3/2, Sum11/2
  Sum3/1 -> Sum/2
  Theta Correction/1 -> Sum7/1, Sum6/2, Sum5/2, Sum/1
  Sum1/1 -> Sum5/1
  Sum8/1 -> Sum6/1
  Sum11/1 -> Sum7/2
  Sum5/1 -> mc1/1
  Sum6/1 -> mc3/1
  Sum7/1 -> mc4/1
  Altitude (z) Correction/1 -> Sum2/1, Sum4/2
  Sum/1 -> mc2/1

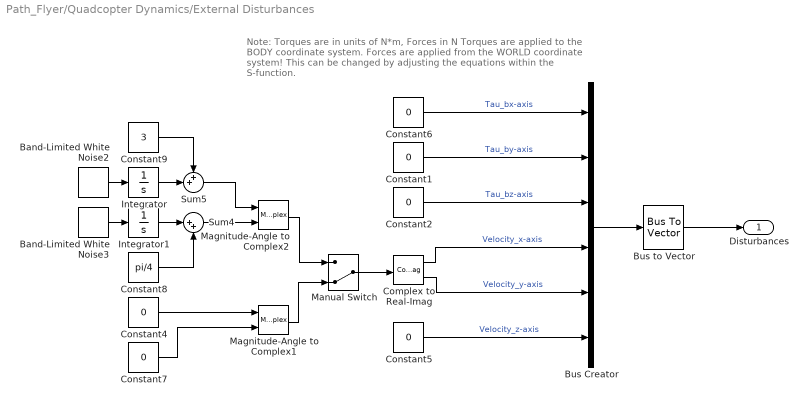
== system Path_Flyer/Quadcopter Dynamics/External Disturbances ==
  note: Note: Torques are in units of N*m, Forces in N
      | Torques are applied to the BODY coordinate system.
      | Forces are applied from the WORLD coordinate system!
      | This can be changed by adjusting the equations within the S-function.
  Band-Limited White Noise2 : simulink/Sources/Band-Limited White Noise  Cov=0.2  Ts=0.1  seed=120516
  Band-Limited White Noise3 : simulink/Sources/Band-Limited White Noise  Cov=0.0025  Ts=0.1  seed=1996
  Bus Creator : BusCreator  Inputs=6
  Bus to Vector : BusToVector
  Complex to Real-Imag : ComplexToRealImag
  Constant{1..2,4..7} (6 alike) : Constant  Value=0
  Constant8 : Constant  Value=pi/4
  Constant9 : Constant  Value=3
  Integrator : Integrator
  Integrator1 : Integrator
  Magnitude-Angle to Complex1 : MagnitudeAngleToComplex
  Magnitude-Angle to Complex2 : MagnitudeAngleToComplex
  Manual Switch : ManualSwitch  CurrentSetting=0
  Sum4 : Sum  Inputs=|++
  Sum5 : Sum  Inputs=++|
  "Disturbances " : Outport
  wires:
  Bus to Vector/1 -> "Disturbances "/1
  Bus Creator/1 -> Bus to Vector/1
  Constant6/1 -> Bus Creator/1  "Tau_bx-axis"
  Constant1/1 -> Bus Creator/2  "Tau_by-axis"
  Constant2/1 -> Bus Creator/3  "Tau_bz-axis"
  Complex to Real-Imag/1 -> Bus Creator/4  "Velocity_x-axis"
  Complex to Real-Imag/2 -> Bus Creator/5  "Velocity_y-axis"
  Constant5/1 -> Bus Creator/6  "Velocity_z-axis"
  Constant4/1 -> Magnitude-Angle to Complex1/1
  Constant7/1 -> Magnitude-Angle to Complex1/2
  Manual Switch/1 -> Complex to Real-Imag/1
  Magnitude-Angle to Complex1/1 -> Manual Switch/2
  Magnitude-Angle to Complex2/1 -> Manual Switch/1
  Sum4/1 -> Magnitude-Angle to Complex2/2
  Sum5/1 -> Magnitude-Angle to Complex2/1
  Constant8/1 -> Sum4/2
  Integrator1/1 -> Sum4/1
  Constant9/1 -> Sum5/1
  Band-Limited White Noise3/1 -> Integrator1/1
  Integrator/1 -> Sum5/2
  Band-Limited White Noise2/1 -> Integrator/1

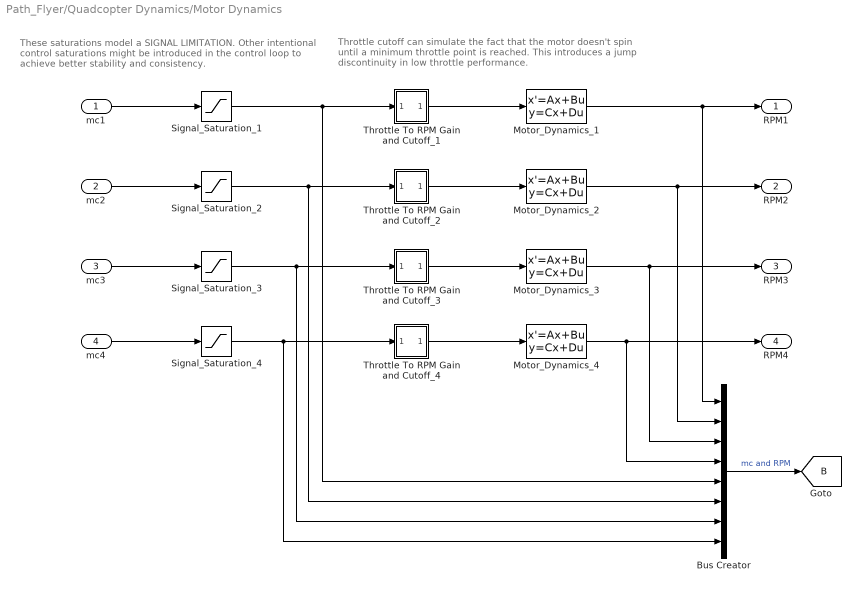
== system Path_Flyer/Quadcopter Dynamics/Motor Dynamics ==
  note: Throttle cutoff can simulate the fact that the motor doesn't
      | spin until a minimum throttle point is reached. This introduces
      | a jump discontinuity in low throttle performance.
  note: These saturations model a SIGNAL LIMITATION.
      | Other intentional control saturations might be introduced in the
      | control loop to achieve better stability and consistency.
  mc1 : Inport
  mc2 : Inport  Port=2
  mc3 : Inport  Port=3
  mc4 : Inport  Port=4
  Bus Creator : BusCreator  Inputs=8
  Motor_Dynamics_1 : StateSpace  A=-1/quadModel.T  C=1/quadModel.T  D=0  InitialCondition=IC.w1*quadModel.T
  Motor_Dynamics_2 : StateSpace  A=-1/quadModel.T  C=1/quadModel.T  D=0  InitialCondition=IC.w2*quadModel.T
  Motor_Dynamics_3 : StateSpace  A=-1/quadModel.T  C=1/quadModel.T  D=0  InitialCondition=IC.w3*quadModel.T
  Motor_Dynamics_4 : StateSpace  A=-1/quadModel.T  C=1/quadModel.T  D=0  InitialCondition=IC.w4*quadModel.T
  Signal_Saturation_{1..4} (4 alike) : Saturate  UpperLimit=200  LowerLimit=1
  Throttle To RPM Gain and Cutoff_1 : Subsystem
  Throttle To RPM Gain and Cutoff_2 : Subsystem
  Throttle To RPM Gain and Cutoff_3 : Subsystem
  Throttle To RPM Gain and Cutoff_4 : Subsystem
  RPM1 : Outport
  RPM2 : Outport  Port=2
  RPM3 : Outport  Port=3
  RPM4 : Outport  Port=4
  tag scope: B=global
  wires:
  mc1/1 -> Signal_Saturation_1/1
  mc4/1 -> Signal_Saturation_4/1
  mc2/1 -> Signal_Saturation_2/1
  mc3/1 -> Signal_Saturation_3/1
  Signal_Saturation_1/1 -> Bus Creator/5, Throttle To RPM Gain and Cutoff_1/1(In5)
  Signal_Saturation_2/1 -> Bus Creator/6, Throttle To RPM Gain and Cutoff_2/1(In5)
  Signal_Saturation_3/1 -> Bus Creator/7, Throttle To RPM Gain and Cutoff_3/1(In5)
  Signal_Saturation_4/1 -> Bus Creator/8, Throttle To RPM Gain and Cutoff_4/1(In5)
  Throttle To RPM Gain and Cutoff_1/1(Out5) -> Motor_Dynamics_1/1
  Throttle To RPM Gain and Cutoff_2/1(Out5) -> Motor_Dynamics_2/1
  Throttle To RPM Gain and Cutoff_3/1(Out5) -> Motor_Dynamics_3/1
  Throttle To RPM Gain and Cutoff_4/1(Out5) -> Motor_Dynamics_4/1
  Motor_Dynamics_1/1 -> Bus Creator/1, RPM1/1
  Motor_Dynamics_2/1 -> Bus Creator/2, RPM2/1
  Motor_Dynamics_3/1 -> Bus Creator/3, RPM3/1
  Motor_Dynamics_4/1 -> Bus Creator/4, RPM4/1
  Bus Creator/1 -> [B]  "mc and RPM"

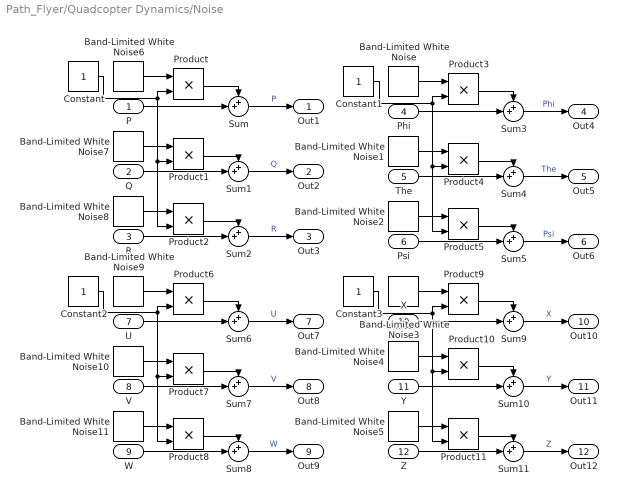
== system Path_Flyer/Quadcopter Dynamics/Noise ==
  P : Inport
  Q : Inport  Port=2
  R : Inport  Port=3
  Phi : Inport  Port=4
  The : Inport  Port=5
  Psi : Inport  Port=6
  U : Inport  Port=7
  V : Inport  Port=8
  W : Inport  Port=9
  X : Inport  Port=10
  Y : Inport  Port=11
  Z : Inport  Port=12
  Band-Limited White Noise : simulink/Sources/Band-Limited White Noise  Cov=(0.01)*1/100*(0.01)*1/100  Ts=1/100  seed=1
  Band-Limited White Noise1 : simulink/Sources/Band-Limited White Noise  Cov=(0.01)*1/100*(0.01)*1/100  Ts=1/100  seed=2
  Band-Limited White Noise10 : simulink/Sources/Band-Limited White Noise  Cov=0.05*0.05*1/5*1/5  Ts=1/5  seed=11
  Band-Limited White Noise11 : simulink/Sources/Band-Limited White Noise  Cov=0.01*0.01*1/100*1/100  Ts=1/100  seed=12
  Band-Limited White Noise2 : simulink/Sources/Band-Limited White Noise  Cov=(0.01)*1/100*(0.01)*1/100  Ts=1/100  seed=3
  Band-Limited White Noise3 : simulink/Sources/Band-Limited White Noise  Cov=0.05*1/5*0.05*1/5  Ts=1/5  seed=4
  Band-Limited White Noise4 : simulink/Sources/Band-Limited White Noise  Cov=0.05*1/5*0.05*1/5  Ts=1/5  seed=5
  Band-Limited White Noise5 : simulink/Sources/Band-Limited White Noise  Cov=0.01*1/100*0.01*1/100  Ts=1/100  seed=6
  Band-Limited White Noise6 : simulink/Sources/Band-Limited White Noise  Cov=0.1*180/pi*1/100*0.1*180/pi*1/100  Ts=1/100  seed=7
  Band-Limited White Noise7 : simulink/Sources/Band-Limited White Noise  Cov=0.1*180/pi*1/100*0.1*180/pi*1/100  Ts=1/100  seed=8
  Band-Limited White Noise8 : simulink/Sources/Band-Limited White Noise  Cov=0.01*180/pi*1/100*0.01*180/pi*1/100  Ts=1/100  seed=9
  Band-Limited White Noise9 : simulink/Sources/Band-Limited White Noise  Cov=0.05*0.05*1/5*1/5  Ts=1/5  seed=10
  Constant{,1..3} (4 alike) : Constant
  Product{,1..11} (12 alike) : Product
  Sum{,1..11} (12 alike) : Sum  Inputs=++|
  Out1 : Outport
  Out2 : Outport  Port=2
  Out3 : Outport  Port=3
  Out4 : Outport  Port=4
  Out5 : Outport  Port=5
  Out6 : Outport  Port=6
  Out7 : Outport  Port=7
  Out8 : Outport  Port=8
  Out9 : Outport  Port=9
  Out10 : Outport  Port=10
  Out11 : Outport  Port=11
  Out12 : Outport  Port=12
  wires:
  P/1 -> Sum/2
  Z/1 -> Sum11/2
  Sum/1 -> Out1/1  "P"
  X/1 -> Sum9/2
  Phi/1 -> Sum3/2
  Sum1/1 -> Out2/1  "Q"
  Q/1 -> Sum1/2
  R/1 -> Sum2/2
  Sum10/1 -> Out11/1  "Y"
  Sum4/1 -> Out5/1  "The"
  The/1 -> Sum4/2
  W/1 -> Sum8/2
  U/1 -> Sum6/2
  Sum2/1 -> Out3/1  "R"
  Psi/1 -> Sum5/2
  Sum9/1 -> Out10/1  "X"
  Sum7/1 -> Out8/1  "V"
  Sum11/1 -> Out12/1  "Z"
  Sum3/1 -> Out4/1  "Phi"
  Y/1 -> Sum10/2
  Sum8/1 -> Out9/1  "W"
  Sum6/1 -> Out7/1  "U"
  Sum5/1 -> Out6/1  "Psi"
  V/1 -> Sum7/2
  Product/1 -> Sum/1
  Band-Limited White Noise6/1 -> Product/1
  Product1/1 -> Sum1/1
  Band-Limited White Noise7/1 -> Product1/1
  Product2/1 -> Sum2/1
  Band-Limited White Noise8/1 -> Product2/1
  Product3/1 -> Sum3/1
  Product4/1 -> Sum4/1
  Band-Limited White Noise1/1 -> Product4/1
  Product5/1 -> Sum5/1
  Band-Limited White Noise2/1 -> Product5/1
  Product6/1 -> Sum6/1
  Band-Limited White Noise9/1 -> Product6/1
  Product7/1 -> Sum7/1
  Band-Limited White Noise10/1 -> Product7/1
  Product8/1 -> Sum8/1
  Band-Limited White Noise11/1 -> Product8/1
  Product9/1 -> Sum9/1
  Band-Limited White Noise3/1 -> Product9/1
  Product10/1 -> Sum10/1
  Band-Limited White Noise4/1 -> Product10/1
  Product11/1 -> Sum11/1
  Band-Limited White Noise5/1 -> Product11/1
  Constant/1 -> Product2/2, Product1/2, Product/2
  Constant1/1 -> Product5/2, Product4/2, Product3/2
  Constant2/1 -> Product6/2, Product8/2, Product7/2
  Constant3/1 -> Product9/2, Product11/2, Product10/2
  Band-Limited White Noise/1 -> Product3/1

== system Path_Flyer/Velocity Controller/Phi Command Control ==
  note: -1 Gain is required because a "negative"
      | angle of Phi induces a positive velocity
      | in the body frame y direction!
  Desired Yb Velocity : Inport
  Yb Velocity : Inport  Port=2
  Attitude Limits_Phi : Saturate  UpperLimit=ASat  LowerLimit=-ASat
  Gain : Gain  Gain=-1
  Kdp : Gain  Gain=Kd
  Kpp : Gain  Gain=Kp
  Sum3 : Sum  Inputs=|+-
  Sum6 : Sum  Inputs=|+-
  V Derivative : Derivative
  Phi_cmd : Outport
  wires:
  V Derivative/1 -> Kdp/1
  Attitude Limits_Phi/1 -> Phi_cmd/1  "Phi_cmd"
  Sum6/1 -> Gain/1
  Kpp/1 -> Sum6/1
  Sum3/1 -> Kpp/1  "Velocity Error"
  Yb Velocity/1 -> V Derivative/1, Sum3/2
  Desired Yb Velocity/1 -> Sum3/1
  Gain/1 -> Attitude Limits_Phi/1
  Kdp/1 -> Sum6/2

== system Path_Flyer/Velocity Controller/Theta Command Control ==
  Desired Xb Velocity : Inport
  Xb Velocity : Inport  Port=2
  Attitude Limits_Theta : Saturate  UpperLimit=ASat  LowerLimit=-ASat
  Kdt : Gain  Gain=Kd
  Kpt : Gain  Gain=Kp
  Sum3 : Sum  Inputs=|+-
  Sum6 : Sum  Inputs=|+-
  U Derivative : Derivative
  The_cmd : Outport
  wires:
  Kdt/1 -> Sum6/2
  U Derivative/1 -> Kdt/1
  Attitude Limits_Theta/1 -> The_cmd/1  "The_cmd"
  Sum6/1 -> Attitude Limits_Theta/1
  Kpt/1 -> Sum6/1
  Sum3/1 -> Kpt/1  "Velocity Error"
  Xb Velocity/1 -> U Derivative/1, Sum3/2
  Desired Xb Velocity/1 -> Sum3/1

== system Path_Flyer/Quadcopter Dynamics/Motor Dynamics/Throttle To RPM Gain and Cutoff_1 ==
  note: minThr should be a quad.mat value
  note: This gain should be a quad.mat value
  note: This constant should be a quad.mat value
  note: Output equals linearly scaled RPM
      | for given throttle input if throttle input >=Throttle Cuttoff (minThr)
      | else output is zero.
  In5 : Inport
  Constant : Constant  Value=quadModel.b
  Gain : Gain  Gain=quadModel.cr
  Minimum Throttle Cutoff : simulink/Logic and Bit Operations/Compare To Constant  relop=>=  const=quadModel.minThr  OutDataTypeStr=uint8
  Product : Product
  Sum1 : Sum  Inputs=++|
  Out5 : Outport
  wires:
  Minimum Throttle Cutoff/1 -> Product/2
  Product/1 -> Out5/1
  In5/1 -> Gain/1, Minimum Throttle Cutoff/1
  Gain/1 -> Sum1/2
  Sum1/1 -> Product/1
  Constant/1 -> Sum1/1

== system Path_Flyer/Quadcopter Dynamics/Motor Dynamics/Throttle To RPM Gain and Cutoff_2 ==
  note: minThr should be a quad.mat value
  note: This gain should be a quad.mat value
  note: This constant should be a quad.mat value
  note: Output equals linearly scaled RPM
      | for given throttle input if throttle input >=Throttle Cuttoff (minThr)
      | else output is zero.
  In5 : Inport
  Constant : Constant  Value=quadModel.b
  Gain : Gain  Gain=quadModel.cr
  Minimum Throttle Cutoff : simulink/Logic and Bit Operations/Compare To Constant  relop=>=  const=quadModel.minThr  OutDataTypeStr=uint8
  Product : Product
  Sum1 : Sum  Inputs=++|
  Out5 : Outport
  wires:
  Minimum Throttle Cutoff/1 -> Product/2
  Product/1 -> Out5/1
  In5/1 -> Gain/1, Minimum Throttle Cutoff/1
  Gain/1 -> Sum1/2
  Sum1/1 -> Product/1
  Constant/1 -> Sum1/1

== system Path_Flyer/Quadcopter Dynamics/Motor Dynamics/Throttle To RPM Gain and Cutoff_3 ==
  note: minThr should be a quad.mat value
  note: This gain should be a quad.mat value
  note: This constant should be a quad.mat value
  note: Output equals linearly scaled RPM
      | for given throttle input if throttle input >=Throttle Cuttoff (minThr)
      | else output is zero.
  In5 : Inport
  Constant : Constant  Value=quadModel.b
  Gain : Gain  Gain=quadModel.cr
  Minimum Throttle Cutoff : simulink/Logic and Bit Operations/Compare To Constant  relop=>=  const=quadModel.minThr  OutDataTypeStr=uint8
  Product : Product
  Sum1 : Sum  Inputs=++|
  Out5 : Outport
  wires:
  Minimum Throttle Cutoff/1 -> Product/2
  Product/1 -> Out5/1
  In5/1 -> Gain/1, Minimum Throttle Cutoff/1
  Gain/1 -> Sum1/2
  Sum1/1 -> Product/1
  Constant/1 -> Sum1/1

== system Path_Flyer/Quadcopter Dynamics/Motor Dynamics/Throttle To RPM Gain and Cutoff_4 ==
  note: minThr should be a quad.mat value
  note: This gain should be a quad.mat value
  note: This constant should be a quad.mat value
  note: Output equals linearly scaled RPM
      | for given throttle input if throttle input >=Throttle Cuttoff (minThr)
      | else output is zero.
  In5 : Inport
  Constant : Constant  Value=quadModel.b
  Gain : Gain  Gain=quadModel.cr
  Minimum Throttle Cutoff : simulink/Logic and Bit Operations/Compare To Constant  relop=>=  const=quadModel.minThr  OutDataTypeStr=uint8
  Product : Product
  Sum1 : Sum  Inputs=++|
  Out5 : Outport
  wires:
  Minimum Throttle Cutoff/1 -> Product/2
  Product/1 -> Out5/1
  In5/1 -> Gain/1, Minimum Throttle Cutoff/1
  Gain/1 -> Sum1/2
  Sum1/1 -> Product/1
  Constant/1 -> Sum1/1
